simulink model "linefollow2"  (R2018b)
settings: Solver=ode3  StartTime=0.0  StopTime=10  RelTol=1e-3
libraries: legoev3lib x3
settings Model: FPTRunName=Active  ExtModeTrigDuration=2  Creator=chris  LastModifiedBy=chris
settings SolverCC: PositivePriorityOrder=on
settings DataIOCC: LimitDataPoints=on  SaveFormat=Array
settings OptimizationCC: ExpressionDepthLimit=2147483647  LifeSpan=Inf  MaxStackSize=64
settings DebuggingCC: UnderspecifiedInitializationDetection=Classic  MergeDetectMultiDrivingBlocksExec=none  FcnCallInpInsideContextMsg=warning  AllowSymbolicDim=off  StateNameClashWarn=warning  SFUnexpectedBacktrackingDiag=warning  SFNoUnconditionalDefaultTransitionDiag=warning  SFExecutionAtInitializationDiag=none
settings HardwareCC: ProdBitPerPointer=32  ProdBitPerSizeT=32  ProdBitPerPtrDiffT=32  ProdLargestAtomicInteger=Long  ProdWordSize=32  ProdHWDeviceType=ARM Compatible->ARM 9  UseEmbeddedCoderFeatures=off  UseSimulinkCoderFeatures=off
settings ModelReferenceCC: PropagateSignalLabelsOutOfModel=off
settings SFSimCC: SimUseLocalCustomCode=off
settings RTWCC: SystemTargetFile=ert.tlc  HardwareBoard=LEGO MINDSTORMS EV3  TemplateMakefile=ert_default_tmf  GenerateReport=on  RTWVerbose=off  RTWUseLocalCustomCode=off  Toolchain=Sourcery G++ Lite v2009q3  BuildConfiguration=Faster Runs  LaunchReport=on
settings CodeAppCC: ForceParamTrailComments=on  OperatorAnnotations=on  StateflowObjectComments=on  MATLABSourceComments=on
settings ERTTargetCC: MultiwordLength=2048  ERTCustomFileBanners=off  SupportContinuousTime=on  SupportNonInlinedSFcns=on  RemoveResetFunc=off  SupportVariableSizeSignals=on  ModelStepFunctionPrototypeControlCompliant=off
settings ConfigComp: CovMetricSettings=dw  CovHtmlReporting=on  CovSaveCumulativeToWorkspaceVar=on  CovSaveSingleToWorkspaceVar=on  CovExternalEMLEnable=off  CovSFcnEnable=off

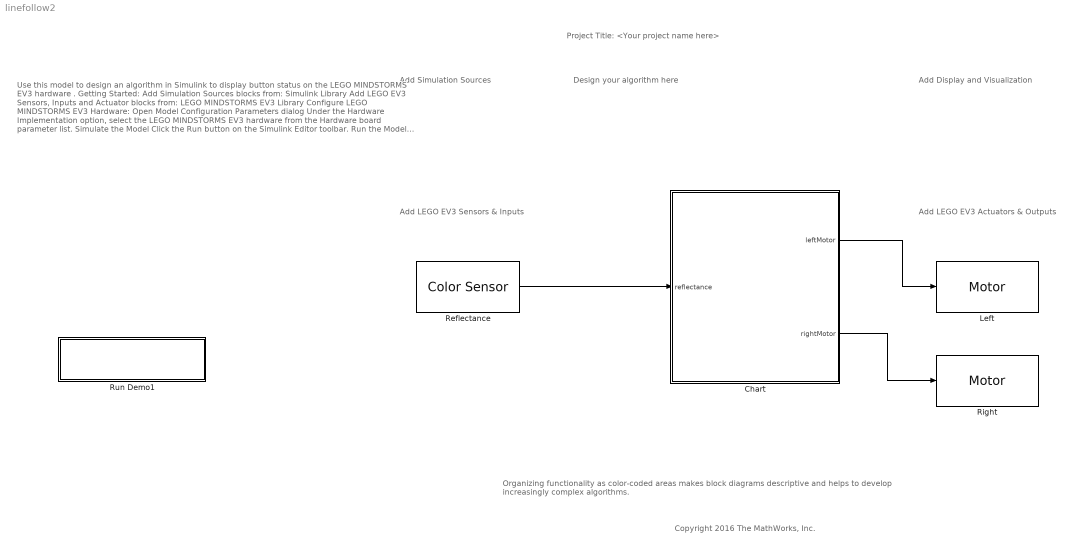
== system linefollow2 ==
  note: Project Title: <Your project name here>
  note: Copyright 2016 The MathWorks, Inc.
  note: Add LEGO EV3 Sensors & Inputs
  note: Add LEGO EV3 Actuators & Outputs
  note: Add Display and Visualization
  note: Design your algorithm here
  note: Add Simulation Sources
  note: Use this model to design an algorithm in Simulink to display button status on the LEGO MINDSTORMS EV3 hardware .
      |
      | Getting Started:
      |
      | Add Simulation Sources blocks from:
      | Simulink Library
      | Add LEGO EV3 Sensors, Inputs and Actuator blocks from:
      | LEGO MINDSTORMS EV3 Library
      |
      | Configure LEGO MINDSTORMS EV3 Hardware:
      |
      | Open Model Configuration Parameters dialog
      | Under the Hardware Implementation option, select the LEGO MINDSTORMS EV3 hardware from the Hardware board parameter list.
      |
      | Simulate the Model
      |
      | Click the Run button on the Simulink Editor toolbar.
      |
      | Run the Model on LEGO MINDSTORMS EV3 Hardware
      |
      | Click the Deploy to Hardware button on the Simulink Editor toolbar.
      |
      | Other Things to Try:
      |
      | Create and run a model that detects the obstacle and stops the LEGO EV3 robot. HINT: Use Ultrasonic Sensor and Motor blocks.
  note: Organizing functionality as color-coded areas makes block diagrams descriptive and helps to develop increasingly complex algorithms.
  Chart : Stateflow chart  TreatAsAtomicUnit=on
  Left : legoev3lib/Motor  sportNumber=C  sstopAction=Brake
  Reflectance : legoev3lib/Color Sensor  portNumber=3  mode=Reflected light intensity  sampleTime=0.001
      settings: SourceProductName=Simulink Support Package for LEGO MINDSTORMS EV3 Hardware  SourceProductBaseCode=LEGOEV3
  Right : legoev3lib/Motor  sportNumber=B  sstopAction=Brake
  Run Demo1 : Subsystem  Description=Controls host-side RTDX processing.
      mask Display: pic=imread('ev3DeploytoHardware.png');image(pic);
  wires:
  Chart/1(leftMotor) -> Left/1
  Reflectance/1 -> Chart/1(reflectance)
  Chart/2(rightMotor) -> Right/1

== system linefollow2/Run Demo1 ==

== stateflow chart linefollow2/Chart ==
  state RecoveryMode
    i = 0
    state Stateymcstateface
      entry:
      reflectanceDeviation = single(reflectance - targetReflectance) / 40;
      i = 0.95 * i + single(reflectanceDeviation);
      rightMotor = driveSpeed - int8(reflectanceDeviation * steerDelta + i * 9.0);
      leftMotor = driveSpeed + int8(reflectanceDeviation * steerDelta + i * 9.0);
    state RecoverToRight
      entry:
      rightMotor = -scanSpeed;
      leftMotor = 2 * scanSpeed;
    state RecoverToLeft
      entry:
      rightMotor = scanSpeed;
      leftMotor = -2 * scanSpeed;
    Stateymcstateface -> Stateymcstateface [order 3] : after(0.01, sec)
    (default) -> Stateymcstateface
    RecoverToRight -> Stateymcstateface : [reflectance < 60]
    Stateymcstateface -> RecoverToRight [order 2] : [reflectance > 60]
    RecoverToLeft -> Stateymcstateface : [reflectance > 10]
    Stateymcstateface -> RecoverToLeft [order 1] : [reflectance < 10]
  (default) -> RecoveryMode
  data: leftMotor output int8; reflectance input uint8; rightMotor output int8; targetReflectance constant uint8 =40; scanSpeed constant int8 =10; driveSpeed constant int8 =40; steerDelta constant single =40; reflectanceDeviation local single; i local single
